simulink model "random_fuzzy"  (R2023a)
settings: Solver=VariableStepAuto  StartTime=0.0  StopTime=1000  RelTol=1e-3
values from neighbouring files (symbols this model uses):
  A1 = 0.0154    [parametros.m]    (also in variables.mat)
  A2 = 5e-5    (= 5e-05)    [parametros.m]    (also in variables.mat)
  az = 0.5    [parametros.m]    (also in variables.mat)
  g = 9.8    [parametros.m]    (also in variables.mat)
  ro = 1000    [parametros.m]    (also in variables.mat)
  semilla = 751    [parametros.m]    (also in variables.mat)
undefined symbols (not defined in the file or in its folder): DiscIntNeverNeededParam
libraries: fuzblock x1
settings Model: Creator=empg0  LastModifiedBy=empg0

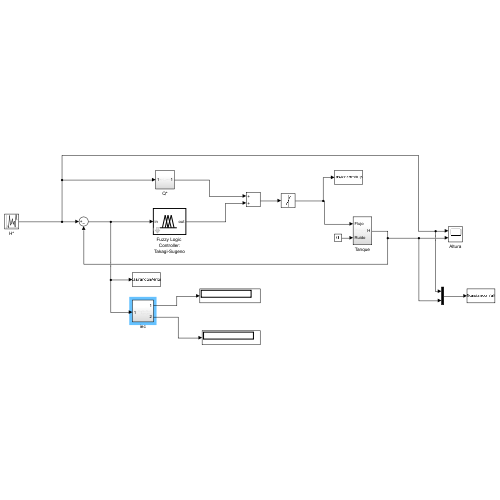
[thumbnail: Simulink's stored preview of the top-level diagram]
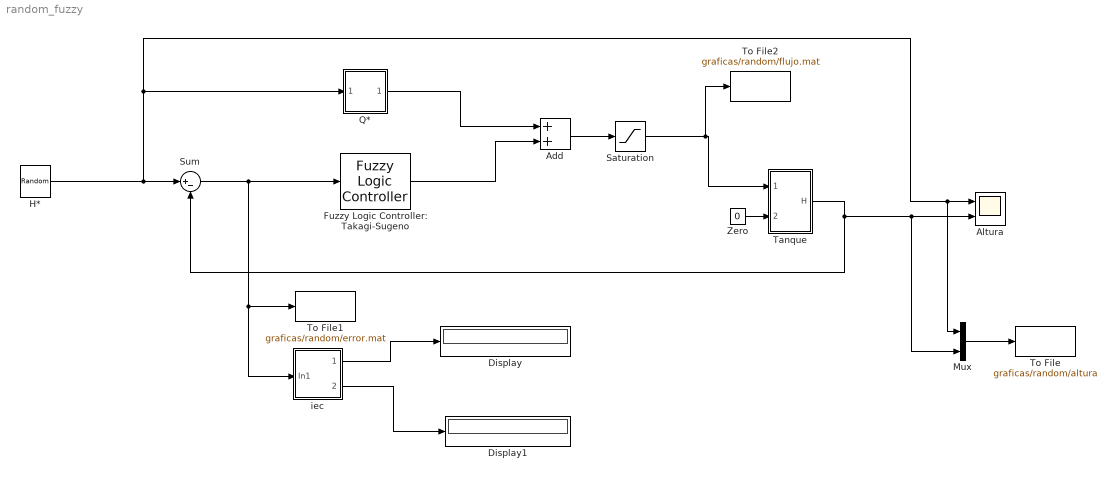
== system random_fuzzy ==
  Add : Sum
  Altura : Scope  NumInputPorts=2
  Display : Display
  Display1 : Display
  Fuzzy Logic Controller: Takagi-Sugeno : fuzblock/Fuzzy Logic  Controller  FIS='error_fuzzy.fis'  OutputSampleNumber=101  DataType=double  FuzzifiedInputs=off  RuleFiringStrengths=off  RuleOutputs=off  AggregatedOutputs=off  SimulateUsing=Interpreted execution  OutOfRangeInputValueMessage=warning  NoRuleFiredMessage=warning  EmptyOutputFuzzySetMessage=warning
  H* : UniformRandomNumber  Minimum=0  Maximum=0.62  Seed=semilla  SampleTime=200
  Mux : Mux  Inputs=2
  Q* : Subsystem
  Saturation : Saturate  UpperLimit=0.1  LowerLimit=0
  Sum : Sum  Inputs=|+-
  Tanque : Subsystem
  To File : ToFile  Filename=graficas/random/altura  MatrixName=altura  SampleTime=0.25
  To File1 : ToFile  Filename=graficas/random/error.mat  MatrixName=error  SampleTime=0.25
  To File2 : ToFile  Filename=graficas/random/flujo.mat  MatrixName=flujo  SampleTime=0.25
  Zero : Constant  Value=0  OutDataTypeStr=Inherit: Inherit via back propagation
  iec : Subsystem
  wires:
  Zero/1 -> Tanque/2(Ruido)
  Tanque/1(H) -> Mux/2, Altura/2, Sum/2
  Sum/1 -> To File1/1, iec/1(In1), Fuzzy Logic Controller: Takagi-Sugeno/1
  Fuzzy Logic Controller: Takagi-Sugeno/1 -> Add/2
  Add/1 -> Saturation/1
  Saturation/1 -> To File2/1, Tanque/1(Flujo)
  H*/1 -> Sum/1, Q*/1(In1), Mux/1, Altura/1
  iec/1(Out1) -> Display/1
  Mux/1 -> To File/1
  Q*/1(Out1) -> Add/1
  iec/2(Out2) -> Display1/1

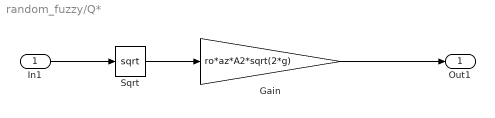
== system random_fuzzy/Q* ==
  In1 : Inport
  Gain : Gain  Gain=ro*az*A2*sqrt(2*g)
  Sqrt : Sqrt
  Out1 : Outport
  wires:
  In1/1 -> Sqrt/1
  Sqrt/1 -> Gain/1
  Gain/1 -> Out1/1

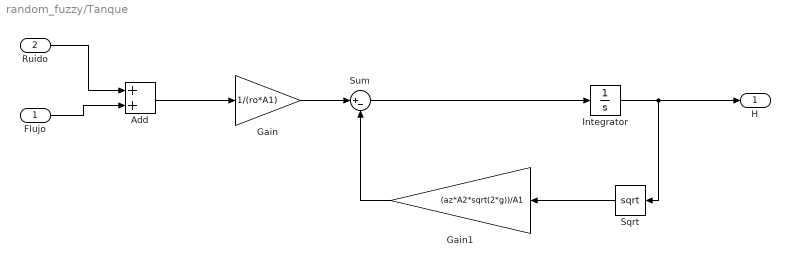
== system random_fuzzy/Tanque ==
  Flujo : Inport
  Ruido : Inport  Port=2
  Add : Sum
  Gain : Gain  Gain=1/(ro*A1)
  Gain1 : Gain  Gain=(az*A2*sqrt(2*g))/A1
  Integrator : Integrator  LimitOutput=on  UpperSaturationLimit=0.62  LowerSaturationLimit=0
  Sqrt : Sqrt
  Sum : Sum  Inputs=|+-
  H : Outport
  wires:
  Gain/1 -> Sum/1
  Sum/1 -> Integrator/1
  Sqrt/1 -> Gain1/1
  Gain1/1 -> Sum/2
  Integrator/1 -> H/1, Sqrt/1
  Add/1 -> Gain/1
  Flujo/1 -> Add/2
  Ruido/1 -> Add/1

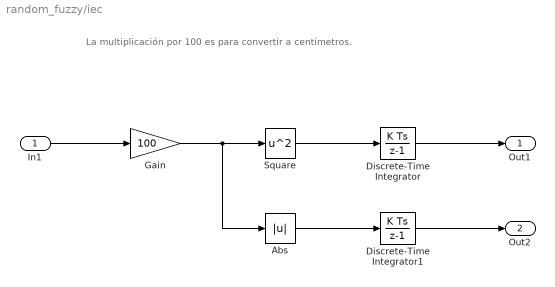
== system random_fuzzy/iec ==
  note: La multiplicación por 100 es para convertir a centímetros.
  In1 : Inport
  Abs : Abs  SaturateOnIntegerOverflow=off
  Discrete-Time Integrator : DiscreteIntegrator  SampleTime=0.001  ICPrevOutput=DiscIntNeverNeededParam  ICPrevScaledInput=DiscIntNeverNeededParam
  Discrete-Time Integrator1 : DiscreteIntegrator  SampleTime=0.001  ICPrevOutput=DiscIntNeverNeededParam  ICPrevScaledInput=DiscIntNeverNeededParam
  Gain : Gain  Gain=100
  Square : Math  Operator=square  SignedPower=on  RndMeth=Zero
  Out1 : Outport
  Out2 : Outport  Port=2
  wires:
  In1/1 -> Gain/1
  Gain/1 -> Abs/1, Square/1
  Square/1 -> Discrete-Time Integrator/1
  Discrete-Time Integrator/1 -> Out1/1
  Discrete-Time Integrator1/1 -> Out2/1
  Abs/1 -> Discrete-Time Integrator1/1
